simulink model "GFLIB_SinCos_BAM_F16"  (Simulink 8.3)
settings: Solver=ode45  StartTime=0.0  StopTime=10.0  RelTol=1e-3
settings Model: Creator=b37097  LastModifiedBy=B17364
settings DataIOCC: SignalLoggingSaveFormat=Dataset
settings DebuggingCC: UnderspecifiedInitializationDetection=Simplified  StateNameClashWarn=none
settings GRTTargetCC: CombineOutputUpdateFcns=on  GRTInterface=off

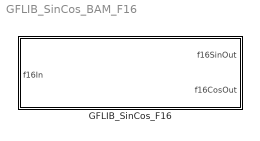
== system GFLIB_SinCos_BAM_F16 ==
  GFLIB_SinCos_F16 : Subsystem  mask(GFLIB_SinCos_F16){}
      mask help: Bit accurate model of GFLIB_SinCos function, which computes the sin(f16In) and cos(f16In) using the 7th order Taylor polynomial approximation.
      mask init:
      | pos = get_param(gcb, 'Position');width = pos(3) - pos(1); height = pos(4) - pos(2);tX=width/2;tY=height*0.9;
      mask Display: color('black');port_label('input',1,'f16In');port_label('output',1,'f16SinOut');port_label('output',2,'f16CosOut');color('black');disp('GFLIB_SinCos_F16');color('blue');text(tX,tY, 'BAM', 'horizontalAlignment', 'center');

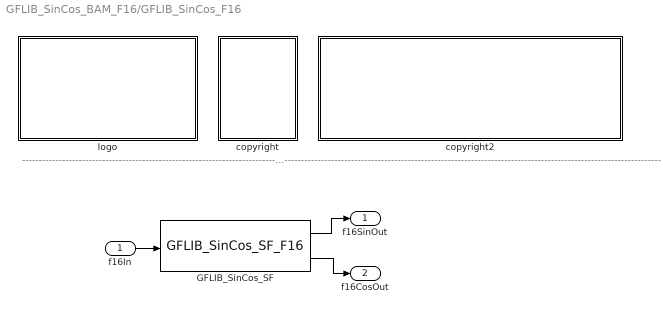
== system GFLIB_SinCos_BAM_F16/GFLIB_SinCos_F16 ==
  note: ---------------------------------------------------------------------------------------------------------------------------------------------------------------------------------------------------
  f16In : Inport
  GFLIB_SinCos_SF : S-Function  FunctionName=GFLIB_SinCos_SF_F16  EnableBusSupport=off
  copyright : Subsystem
      mask Display: text(10,90,'FILE:');text(10,75,'DESRIPTION:');text(10,60,'COPYRIGHT:');text(10,45,'VERSION:');text(10,30,'DATE:')
  copyright2 : Subsystem
      mask Display: text(10,90,'GFLIB_SinCos_BAM_F16.mdl');text(10,75,'Sine and Cosine transformation');text(10,60,'Freescale');text(10,45,'0.1');text(10,30,'27-Sep-2015');
  logo : Subsystem
      mask Display: image(imread('logo.jpg'))
  f16SinOut : Outport
  f16CosOut : Outport  Port=2
  wires:
  f16In/1 -> GFLIB_SinCos_SF/1
  GFLIB_SinCos_SF/1 -> f16SinOut/1
  GFLIB_SinCos_SF/2 -> f16CosOut/1

== system GFLIB_SinCos_BAM_F16/GFLIB_SinCos_F16/copyright ==

== system GFLIB_SinCos_BAM_F16/GFLIB_SinCos_F16/copyright2 ==

== system GFLIB_SinCos_BAM_F16/GFLIB_SinCos_F16/logo ==
